simulink model "Topic_6"  (R2016a)
settings: Solver=FixedStepDiscrete  StartTime=0.0  StopTime=inf  RelTol=1e-3
libraries: simulink x1
settings Model: Creator=yasme  LastModifiedBy=yasme
settings OptimizationCC: DefaultParameterBehavior=Inlined  OptimizeModelRefInitCode=on  LifeSpan=1
settings DebuggingCC: UnderspecifiedInitializationDetection=Classic  MergeDetectMultiDrivingBlocksExec=none
settings ModelReferenceCC: PropagateSignalLabelsOutOfModel=off
settings RTWCC: SystemTargetFile=ert.tlc  GenCodeOnly=on  TemplateMakefile=ert_default_tmf  GenerateReport=on  IncludeHyperlinkInReport=on  LaunchReport=on  GenerateTraceInfo=on  GenerateTraceReport=on  GenerateTraceReportSl=on  GenerateTraceReportSf=on  GenerateTraceReportEml=on
settings CodeAppCC: ForceParamTrailComments=on  IgnoreCustomStorageClasses=off  OperatorAnnotations=on  SimulinkDataObjDesc=on  SFDataObjDesc=on  MATLABFcnDesc=on  InsertBlockDesc=on  MATLABSourceComments=on
settings ERTTargetCC: GenerateSampleERTMain=on  InlinedParameterPlacement=NonHierarchical  ERTCustomFileTemplate=example_file_process.tlc

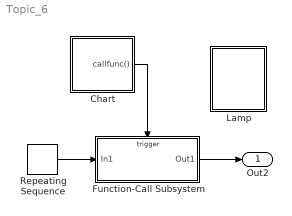
== system Topic_6 ==
  Chart : Stateflow chart  TreatAsAtomicUnit=on
  Function-Call Subsystem : Subsystem  TreatAsAtomicUnit=on
  Lamp : Subsystem  DialogController=hmiCreateDDGDialog  IsWebBlock=on  mask(MWDashboardBlock){webBlockId=270aa6e6-eb5d-44ed-ba05-3a2a4bedc3bd, webBlockType=lamp, ShowInLibBrowser=on, ShowInitialText=on, HMISrcModelName=Topic_6}
      mask prompts: webBlockType "WebBlock Type"; HMISrcModelName "Source Model"
      mask Help: helpview([docroot '/mapfiles/simulink.map'], 'hmi_lamp')
      mask Display:
      | if strcmp(get_param(bdroot(gcb),'BlockDiagramType'), 'library')
      |     image([(matlabroot) '/toolbox/simulink/hmi/icons/Lamp.png']);
      | end
  Repeating Sequence : simulink/Sources/Repeating Sequence  rep_seq_t=[0 0.5 1 1.5 2 2.5]  rep_seq_y=[0 1 0 1 0 1]
  Out2 : Outport
  wires:
  Function-Call Subsystem/1(Out1) -> Out2/1
  Chart/1(callfunc()) -> Function-Call Subsystem/Trigger
  Repeating Sequence/1 -> Function-Call Subsystem/1(In1)

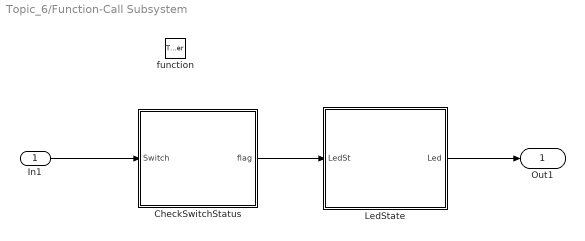
== system Topic_6/Function-Call Subsystem ==
  In1 : Inport
  function : TriggerPort  TriggerType=function-call  VariantControl=Variant
  CheckSwitchStatus : Stateflow chart  TreatAsAtomicUnit=on
  LedState : Stateflow chart  TreatAsAtomicUnit=on
  Out1 : Outport
  wires:
  In1/1 -> CheckSwitchStatus/1(Switch)
  CheckSwitchStatus/1(flag) -> LedState/1(LedSt)
  LedState/1(Led) -> Out1/1

== system Topic_6/Lamp ==

== stateflow chart Topic_6/Function-Call Subsystem/LedState ==
  (default) -> (junction 7) : % LecState
  (junction 7) -> (junction 8) [order 1] : [LedSt==1]
  (junction 7) -> (junction 9) [order 2] : {Led=0;}
  (junction 8) -> (junction 10) : {Led=1;}
  (junction 10) -> (junction 9)
  (junction 9) -> (junction 11)
  data: LedSt input; Led output

== stateflow chart Topic_6/Chart ==
  state call
    en:
    du:
    ex:
  (default) -> call
  call -> call : [after(10,msec)]{callfunc;}
  events: callfunc output FUNCTION_CALL_EVENT

== stateflow chart Topic_6/Function-Call Subsystem/CheckSwitchStatus ==
  (default) -> (junction 7) : % Check Button
  (junction 7) -> (junction 8) [order 1] : [Switch==1]
  (junction 7) -> (junction 9) [order 2] : {flag=0;}
  (junction 8) -> (junction 10) : {flag=1;}
  (junction 10) -> (junction 9)
  (junction 9) -> (junction 11)
  data: Switch input; flag output
